simulink model "Parameters"  (R2020a)
settings: Solver=FixedStepAuto  StartTime=0.0  StopTime=10.0  FixedStep=1e-3  RelTol=1e-3  EnableMultiTasking=on
settings Model: ExtModeTrigDuration=5  Creator=Liam  LastModifiedBy=WinnieTrandinh
settings OptimizationCC: EnhancedBackFolding=on  PassReuseOutputArgsAs=Individual arguments  ZeroExternalMemoryAtStartup=off  ZeroInternalMemoryAtStartup=off  MaxStackSize=64  OptimizeBlockOrder=speed  DifferentSizesBufferReuse=on  OptimizationCustomize=off  EfficientTunableParamExpr=on
settings DebuggingCC: ParameterTunabilityLossMsg=error
settings HardwareCC: ProdBitPerPointer=32  ProdBitPerSizeT=32  ProdBitPerPtrDiffT=32  ProdLargestAtomicInteger=Long  ProdLargestAtomicFloat=Double  ProdWordSize=32  ProdHWDeviceType=ARM Compatible->ARM Cortex
settings SFSimCC: MATLABDynamicMemAlloc=off
settings RTWCC: SystemTargetFile=ert.tlc  HardwareBoard=NXP FRDM-K64F  TemplateMakefile=ert_default_tmf  Toolchain=GNU Tools for ARM Embedded Processors
settings CodeAppCC: ForceParamTrailComments=on  IgnoreCustomStorageClasses=off  OperatorAnnotations=on  SimulinkDataObjDesc=on  SFDataObjDesc=on  InsertBlockDesc=on

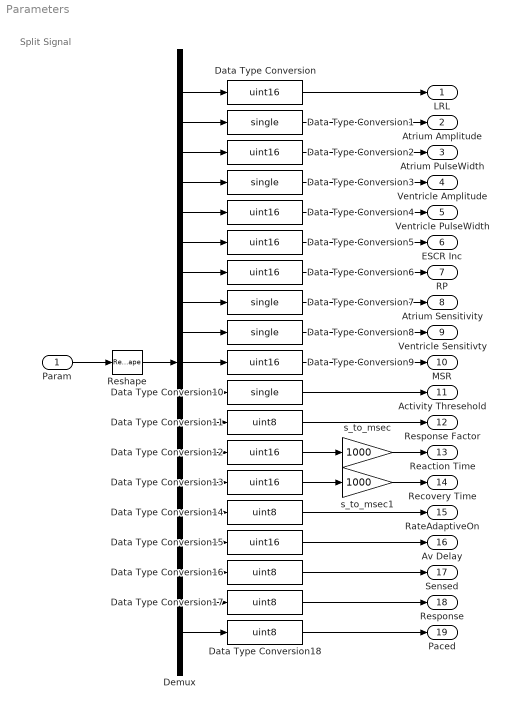
== system Parameters ==
  note: Split Signal
  Param : Inport  OutDataTypeStr=single
  Data Type Conversion{,2,4..6,9,12..13,15} (9 alike) : DataTypeConversion  OutDataTypeStr=uint16
  Data Type Conversion{1,3,7..8,10} (5 alike) : DataTypeConversion  OutDataTypeStr=single
  Data Type Conversion{11,14,16..18} (5 alike) : DataTypeConversion  OutDataTypeStr=uint8
  Demux : Demux  Outputs=19
  Reshape : Reshape  OutputDimensionality=Column vector (2-D)
  s_to_msec : Gain  Gain=1000
  s_to_msec1 : Gain  Gain=1000
  LRL : Outport
  "Atrium Amplitude " : Outport  Port=2
  Atrium PulseWidth : Outport  Port=3
  Ventricle Amplitude : Outport  Port=4
  "Ventricle PulseWidth " : Outport  Port=5
  ESCR Inc : Outport  Port=6
  RP : Outport  Port=7
  "Atrium Sensitivity " : Outport  Port=8
  Ventricle Sensitivty : Outport  Port=9
  MSR : Outport  Port=10
  Activity Thresehold : Outport  Port=11
  Response Factor : Outport  Port=12
  Reaction Time : Outport  Port=13
  Recovery Time : Outport  Port=14
  RateAdaptiveOn : Outport  Port=15
  Av Delay : Outport  Port=16
  Sensed : Outport  Port=17
  Response : Outport  Port=18
  Paced : Outport  Port=19
  wires:
  Demux/1 -> Data Type Conversion/1
  Demux/2 -> Data Type Conversion1/1
  Demux/3 -> Data Type Conversion2/1
  Demux/4 -> Data Type Conversion3/1
  Demux/5 -> Data Type Conversion4/1
  Demux/6 -> Data Type Conversion5/1
  Demux/7 -> Data Type Conversion6/1
  Demux/8 -> Data Type Conversion7/1
  Demux/9 -> Data Type Conversion8/1
  Demux/10 -> Data Type Conversion9/1
  Demux/11 -> Data Type Conversion10/1
  Demux/12 -> Data Type Conversion11/1
  Demux/13 -> Data Type Conversion12/1
  Demux/14 -> Data Type Conversion13/1
  Demux/15 -> Data Type Conversion14/1
  Demux/16 -> Data Type Conversion15/1
  Demux/17 -> Data Type Conversion16/1
  Demux/18 -> Data Type Conversion17/1
  Demux/19 -> Data Type Conversion18/1
  Param/1 -> Reshape/1
  Data Type Conversion/1 -> LRL/1
  Data Type Conversion2/1 -> Atrium PulseWidth/1
  Data Type Conversion5/1 -> ESCR Inc/1
  Data Type Conversion6/1 -> RP/1
  Data Type Conversion8/1 -> Ventricle Sensitivty/1
  Data Type Conversion9/1 -> MSR/1
  Data Type Conversion10/1 -> Activity Thresehold/1
  Data Type Conversion11/1 -> Response Factor/1
  Data Type Conversion12/1 -> s_to_msec/1
  Data Type Conversion13/1 -> s_to_msec1/1
  Data Type Conversion14/1 -> RateAdaptiveOn/1
  Data Type Conversion15/1 -> Av Delay/1
  Data Type Conversion16/1 -> Sensed/1
  Data Type Conversion17/1 -> Response/1
  Data Type Conversion18/1 -> Paced/1
  Reshape/1 -> Demux/1
  Data Type Conversion1/1 -> "Atrium Amplitude "/1
  Data Type Conversion4/1 -> "Ventricle PulseWidth "/1
  Data Type Conversion3/1 -> Ventricle Amplitude/1
  Data Type Conversion7/1 -> "Atrium Sensitivity "/1
  s_to_msec/1 -> Reaction Time/1
  s_to_msec1/1 -> Recovery Time/1
